simulink model "fullorderobserver"  (R2020a)
settings: Solver=VariableStepAuto  StartTime=0.0  StopTime=0.04  RelTol=1e-3
values from neighbouring files (symbols this model uses):
  A = [-6.30908 0 -10.9544 0 83.74458 0 0 24.05866 ... (first row only)    [project2.m]
  Aobs = A - K*C    [project2.m]
  B = BT'    [project2.m]
  Bobs = [B K]    [project2.m]
  C = [0 0 0 5.066579 -116.446 0 0 0 ... (first row only)    [project2.m]
  Cobs = eye(n)    [project2.m]
  D = zeros(c, m)    [project2.m]
  Dobs = zeros(n, m+c)    [project2.m]
  F = place(A, B, dpoles)    [project2.m]
  x0 = [1 2 3 4 5 6 7 8]'    [project2.m]
  x0hat = pinv(C'*C)*C'*y0    [project2.m]
settings Model: Creator=Alan  LastModifiedBy=Alan

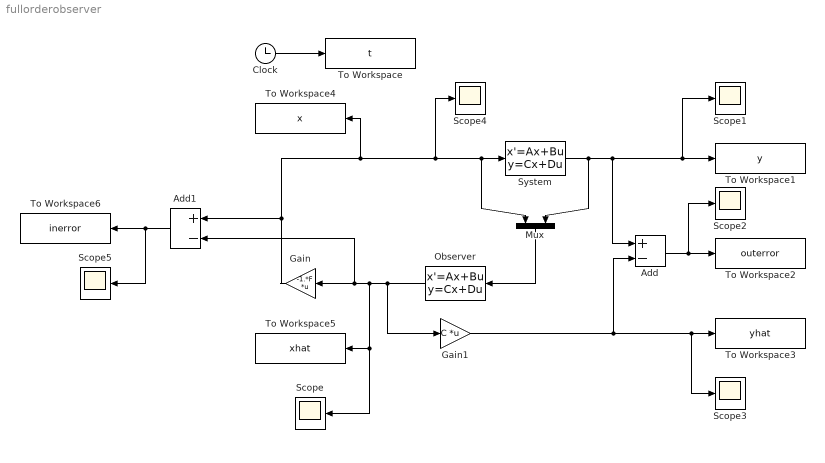
== system fullorderobserver ==
  Add : Sum  Inputs=+-
  Add1 : Sum  Inputs=+-
  Clock : Clock
  Gain : Gain  Gain=-1.*F  Multiplication=Matrix(K*u)
  Gain1 : Gain  Gain=C  Multiplication=Matrix(K*u)
  Mux : Mux  Inputs=2
  Observer : StateSpace  A=Aobs  B=Bobs  C=Cobs  D=Dobs  InitialCondition=x0hat
  Scope{,1..5} (6 alike) : Scope
  System : StateSpace  A=A  B=B  C=C  D=D  InitialCondition=x0
  To Workspace : ToWorkspace  VariableName=t  SaveFormat=Timeseries  SampleTime=-1
  To Workspace1 : ToWorkspace  VariableName=y  SaveFormat=Timeseries  SampleTime=-1
  To Workspace2 : ToWorkspace  VariableName=outerror  SaveFormat=Timeseries  SampleTime=-1
  To Workspace3 : ToWorkspace  VariableName=yhat  SaveFormat=Timeseries  SampleTime=-1
  To Workspace4 : ToWorkspace  VariableName=x  SaveFormat=Timeseries  SampleTime=-1
  To Workspace5 : ToWorkspace  VariableName=xhat  SaveFormat=Timeseries  SampleTime=-1
  To Workspace6 : ToWorkspace  VariableName=inerror  SaveFormat=Timeseries  SampleTime=-1
  wires:
  Clock/1 -> To Workspace/1
  Gain/1 -> To Workspace4/1, Scope4/1, Mux/1, System/1, Add1/1
  Observer/1 -> Gain1/1, Add1/2, Gain/1, To Workspace5/1, Scope/1
  Mux/1 -> Observer/1
  System/1 -> Mux/2, Scope1/1, To Workspace1/1, Add/1
  Gain1/1 -> Scope3/1, To Workspace3/1, Add/2
  Add/1 -> Scope2/1, To Workspace2/1
  Add1/1 -> Scope5/1, To Workspace6/1
